simulink model "linmodel_eq2"  (R2019a)
settings: Solver=VariableStepAuto  StartTime=0.0  StopTime=10.0  RelTol=1e-3
undefined symbols (not defined in the file or in its folder): matrcomp, par
settings Model: Creator=jessi  LastModifiedBy=jessi

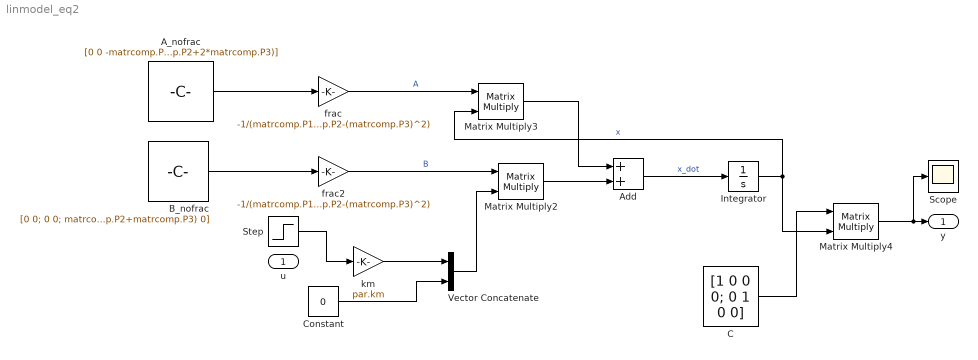
== system linmodel_eq2 ==
  u : Inport
  A_nofrac : Constant  Value=|
      | [0 0 -matrcomp.P1*matrcomp.P2+(matrcomp.P3)^2 0; 0 0 0 -matrcomp.P1*matrcomp.P2+(matrcomp.P3)^2; matrcomp.g1*matrcomp.P2-matrcomp.g2*matrcomp.P3 -matrcomp.g2*matrcomp.P3 par.b1*matrcomp.P2 -par.b2*(matrcomp.P2+matrcomp.P3);
      |              -matrcomp.g1*(matrcomp.P2+matrcomp.P3)+matrcomp.g2*(matrcomp.P1+matrcomp.P3) matrcomp.g2*(matrcomp.P1+matrcomp.P3) -par.b1*(matrcomp.P2+matrcomp.P3) par.b2*(matrcomp.P1+matrcomp.P2+2*matrcomp.P3)]
  Add : Sum
  B_nofrac : Constant  Value=[0 0; 0 0; matrcomp.P2*par.km 0; -par.km*(matrcomp.P2+matrcomp.P3) 0]
  C : Constant  Value=|
      | [1 0 0 0;
      | 0 1 0 0]
  Constant : Constant  Value=0
  Integrator : Integrator
  Matrix Multiply2 : Product  Multiplication=Matrix(*)
  Matrix Multiply3 : Product  Multiplication=Matrix(*)
  Matrix Multiply4 : Product  Multiplication=Matrix(*)
  Scope : Scope
  Step : Step  Time=0.3  SampleTime=0
  Vector Concatenate : Concatenate
  frac : Gain  Gain=-1/(matrcomp.P1*matrcomp.P2-(matrcomp.P3)^2)
  frac2 : Gain  Gain=-1/(matrcomp.P1*matrcomp.P2-(matrcomp.P3)^2)
  km : Gain  Gain=par.km
  y : Outport
  wires:
  frac2/1 -> Matrix Multiply2/1  "B"
  Matrix Multiply2/1 -> Add/2
  frac/1 -> Matrix Multiply3/1  "A"
  Add/1 -> Integrator/1  "x_dot"
  Integrator/1 -> Matrix Multiply4/2, Matrix Multiply3/2  "x"
  Matrix Multiply3/1 -> Add/1
  Matrix Multiply4/1 -> Scope/1, y/1
  A_nofrac/1 -> frac/1
  B_nofrac/1 -> frac2/1
  km/1 -> Vector Concatenate/1
  Constant/1 -> Vector Concatenate/2
  Vector Concatenate/1 -> Matrix Multiply2/2
  C/1 -> Matrix Multiply4/1
  Step/1 -> km/1
